simulink model "ReferBlocks"  (R2015b)
settings: Solver=VariableStepAuto  StartTime=0.0  StopTime=10.0  RelTol=1e-3
settings Model: Creator=sysla  LastModifiedBy=sysla

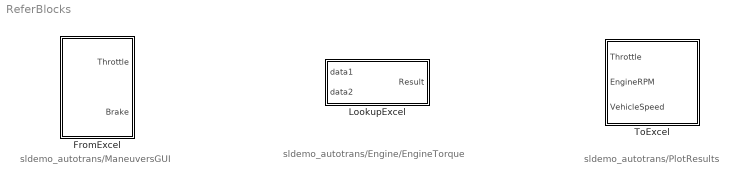
== system ReferBlocks ==
  note: sldemo_autotrans/ManeuversGUI
  note: sldemo_autotrans/PlotResults
  note: sldemo_autotrans/Engine/EngineTorque
  FromExcel : Subsystem  mask{ShowInLibBrowser=on}
      settings: CopyFcn=set_param(gcb,'LinkStatus','none');  OpenFcn=FromExcelGUI(gcb);
  LookupExcel : Subsystem  mask{ShowInLibBrowser=on}
      settings: CopyFcn=set_param(gcb,'LinkStatus','none');  OpenFcn=LookupExcelGUI(gcb);
  ToExcel : Subsystem  StopFcn=|  mask{ShowInLibBrowser=on}
      | guiData = get_param(gcb,'UserData');
      | try
      | writeToExcel(guiData);
      | catch
      | 
      | end
      settings: CopyFcn=set_param(gcb,'LinkStatus','none');  OpenFcn=ToExcelGUI(gcb);

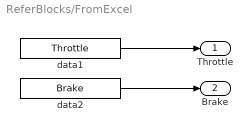
== system ReferBlocks/FromExcel ==
  data1 : FromWorkspace  VariableName=Throttle  SampleTime=0
  data2 : FromWorkspace  VariableName=Brake  SampleTime=0
  Throttle : Outport
  Brake : Outport  Port=2
  wires:
  data1/1 -> Throttle/1
  data2/1 -> Brake/1

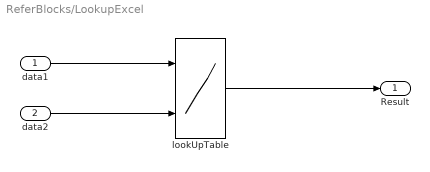
== system ReferBlocks/LookupExcel ==
  data1 : Inport
  data2 : Inport  Port=2
  lookUpTable : Lookup_n-D  BreakpointsForDimension1=[0;20;30;40;50;60;70;80;90;100]  BreakpointsForDimension2=[800 1200 1600 2000 2400 2800 3200 3600 4000 4400 4800]  BreakpointsForDimension3=[5, 7]  Table=[-40 -44 -49 -53 -57 -61 -65 -70 -74 -78 -82;215 117 85 66 44 29 10 -2 -13 -22 -32;245 208 178 148 122 104 85 66 48 33 18;264 260 241 219 193 167 152 133 119 96 85;264 279 282 275 260 238 223 208 189 171 152;267 290 293 297 290 275 260 256 234 212 193;267 297 305 305 305 301 293 282 267 249 226;267 301 308 312 319 323 319 316 297 279 253;267 301 312 319 327 327 327 327 312 293 267;267 301 312 319 327 334 334 334 319 305 275]  InternalRulePriority=Speed  RndMeth=Simplest  InputSameDT=on
  Result : Outport
  wires:
  data1/1 -> lookUpTable/1
  data2/1 -> lookUpTable/2
  lookUpTable/1 -> Result/1

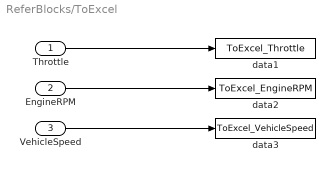
== system ReferBlocks/ToExcel ==
  Throttle : Inport
  EngineRPM : Inport  Port=2
  VehicleSpeed : Inport  Port=3
  data1 : ToWorkspace  VariableName=ToExcel_Throttle  SaveFormat=Timeseries  SampleTime=-1
  data2 : ToWorkspace  VariableName=ToExcel_EngineRPM  SaveFormat=Timeseries  SampleTime=-1
  data3 : ToWorkspace  VariableName=ToExcel_VehicleSpeed  SaveFormat=Timeseries  SampleTime=-1
  wires:
  Throttle/1 -> data1/1
  EngineRPM/1 -> data2/1
  VehicleSpeed/1 -> data3/1
